simulink model "ch5example1"  (Simulink 5.0)
settings: Solver=ode5  StartTime=0.0  StopTime=10.0  FixedStep=6.23e-8  RelTol=1e-3
libraries: dsparch4 x3, dspstat3 x1, dspmathops x1
settings Model: LastModifiedBy=lenovo

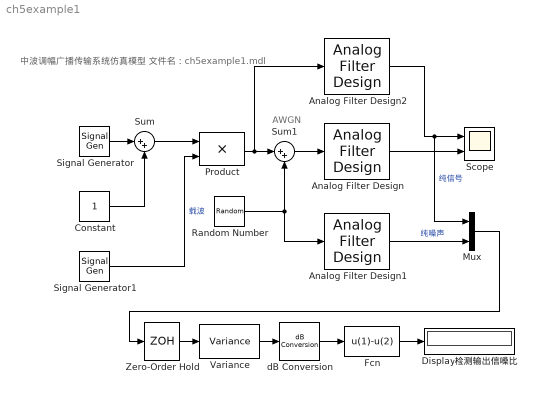
== system ch5example1 ==
  note: 中波调幅广播传输系统仿真模型
      | 文件名：ch5example1.mdl
  note: AWGN
  Analog Filter Design : dsparch4/Analog Filter Design  method=Butterworth  filttype=Bandpass  N=2  Wlo=2*pi*(1e6-6e3)  Whi=2*pi*(1e6+6e3)  Rp=2  Rs=40
  Analog Filter Design1 : dsparch4/Analog Filter Design  method=Butterworth  filttype=Bandpass  N=4  Wlo=2*pi*(1e6-6e3)  Whi=2*pi*(1e6+6e3)  Rp=2  Rs=40
  Analog Filter Design2 : dsparch4/Analog Filter Design  method=Butterworth  filttype=Bandpass  N=4  Wlo=2*pi*(1e6-6e3)  Whi=2*pi*(1e6+6e3)  Rp=2  Rs=40
  Constant : Constant
  Display检测输出信噪比 : Display
  Fcn : Fcn  Expr=u(1)-u(2)
  Mux : Mux  Inputs=2
  Product : Product  SaturateOnIntegerOverflow=on
  Random Number : RandomNumber  Variance=3.4945  SampleTime=6.23e-8
  Scope : Scope  NumInputPorts=2
      settings: TimeRange=0.005  YMin=-1.5~-2  YMax=1.5~2
  Signal Generator : SignalGenerator  Amplitude=0.3  Frequency=1000
  Signal Generator1 : SignalGenerator  Frequency=1000e3
  Sum : Sum  Inputs=|++  SaturateOnIntegerOverflow=on
  Sum1 : Sum  Inputs=|++  SaturateOnIntegerOverflow=on
  Variance : dspstat3/Variance  run=on  reset_popup=None
  Zero-Order Hold : ZeroOrderHold  SampleTime=6.23e-8
  dB Conversion : dspmathops/dB Conversion  dBtype=dB  intype=Power  R=1  fuzz=on
  wires:
  Constant/1 -> Sum/2
  Signal Generator/1 -> Sum/1
  Zero-Order Hold/1 -> Variance/1
  Sum/1 -> Product/1
  Signal Generator1/1 -> Product/2  "载波"
  Product/1 -> Sum1/1, Analog Filter Design2/1
  Random Number/1 -> Sum1/2, Analog Filter Design1/1
  Sum1/1 -> Analog Filter Design/1
  Analog Filter Design/1 -> Scope/2
  Variance/1 -> dB Conversion/1
  dB Conversion/1 -> Fcn/1
  Analog Filter Design1/1 -> Mux/2  "纯噪声"
  Analog Filter Design2/1 -> Scope/1, Mux/1  "纯信号"
  Fcn/1 -> Display检测输出信噪比/1
  Mux/1 -> Zero-Order Hold/1
